simulink library "vil"  (Simulink 8.1)
settings: Solver=ode1  StartTime=0.0  StopTime=Inf  FixedStep=0.001  RelTol=1e-3
PostLoadFcn:
  | , if any(exist('dsrtsu_mdlpostloadfcn', 'file') == [2, 3, 6]), try dsrtsu_mdlpostloadfcn('Execute', bdroot); catch fprintf('Error in PostLoadFcn (dsrtsu_mdlpostloadfcn) for model "%s":\n %s\n', bdroot, lasterr); end, end,
undefined symbols (not defined in the file or in its folder): KIFO_VILOffsetToBumper_m
libraries: hcu_lib x1
settings Model: DSRTSU_INTERNAL_RTI_VER=450  DSRTSU_INTERNAL_RTI_TYPE=rti1401  RTICANMMDATA=struct('GeneralSetupData',struct('modelroot','D:\ELN150201_TAIWAN\trunk\AdasDragon\software\sw_development\arch\app\ifo','generalsettings',struct('filesettings',struct('destfolder',struct('Name','RTICANMM_FILES','Check',1),'buildfolder',struct('Name','.','Check',1),'AbsDestfolder',struct('Name','D:\ELN150201_TAIWAN\trunk\AdasDragon\software\sw_development\arch\app\ifo\RTICANMM_FILES'),'AbsBuildfolder',struct('Name','D:\ELN150201_TAIWAN\trunk\AdasDragon\software\sw_development\arch\app\ifo'))),'options',struct('addpaths',1,'rmpaths',1,'addtrcexclusion',logical(1),'cannavigator',struct('checkmonitoring',0),'show_usrtrc',0,'use_usrtrc',0),'advanced',struct('options',[1 1 1 1 1 1 1 1 1 1 1 1 1 1 1 1 1 1 1 1 1 1 1 1 1 1 1 1 1 1 1 1 1 1 1 1 1 1 1 1 1 1 1 1 1 1 1 1 1 1 1 1 1 1 1 1 1 1 1 1 1 1 1 1 1 1 1 1 1 1 1 1 1 1 1 1 1 1 1 1 1 1 1 1 1 1 1 1 1 1 1 1 1 1 1 1 1 1 1 1]),'MPSetup',{{}},'modelname','vil','block','vil'))  DSRTSU_INTERNAL_RTIFPGA=40  Creator=tescamilla  LastModifiedBy=AT015555

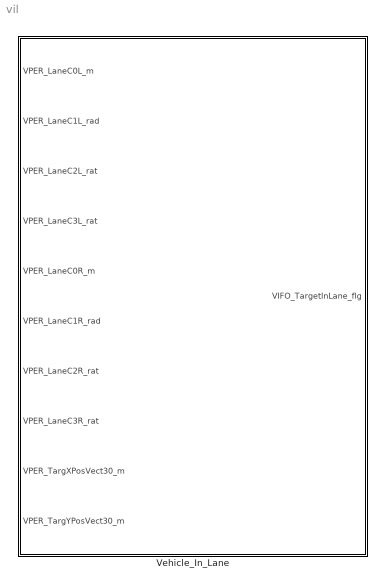
== system vil ==
  Vehicle_In_Lane : Subsystem

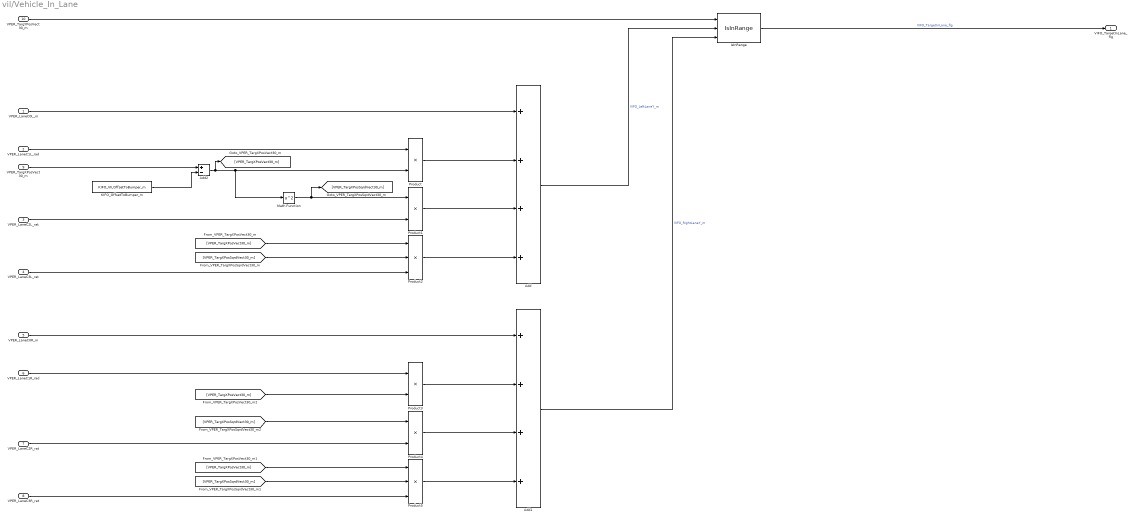
== system vil/Vehicle_In_Lane ==
  VPER_LaneC0L_m : Inport
  VPER_LaneC1L_rad : Inport  Port=2
  VPER_LaneC2L_rat : Inport  Port=3
  VPER_LaneC3L_rat : Inport  Port=4
  VPER_LaneC0R_m : Inport  Port=5
  VPER_LaneC1R_rad : Inport  Port=6
  VPER_LaneC2R_rat : Inport  Port=7
  VPER_LaneC3R_rat : Inport  Port=8
  VPER_TargXPosVect30_m : Inport  Port=9
  VPER_TargYPosVect30_m : Inport  Port=10
  Add : Sum  Inputs=++++
  Add1 : Sum  Inputs=++++
  Add2 : Sum  Inputs=+-
  IsInRange : hcu_lib/IsInRange  SystemSampleTime=-1
  KIFO_OffsetToBumper_m : Constant  Value=KIFO_VILOffsetToBumper_m
  Math Function : Math  Operator=square  SaturateOnIntegerOverflow=on
  Product{,1,3..4} (4 alike) : Product
  Product2 : Product  Inputs=3
  Product5 : Product  Inputs=3
  VIFO_TargetInLane_flg : Outport
  wires:
  VPER_LaneC1L_rad/1 -> Product/1
  Add2/1 -> [VPER_TargXPosVect30_m], Math Function/1, Product/2
  VPER_LaneC0L_m/1 -> Add/1
  Product/1 -> Add/2
  [VPER_TargXPosSqrdVect30_m] -> Product2/2
  VPER_LaneC2L_rat/1 -> Product1/2
  Product1/1 -> Add/3
  Math Function/1 -> [VPER_TargXPosSqrdVect30_m], Product1/1
  [VPER_TargXPosVect30_m] -> Product2/1
  VPER_LaneC3L_rat/1 -> Product2/3
  Product2/1 -> Add/4
  Add/1 -> IsInRange/2  "VIFO_LeftLaneY_m"
  VPER_LaneC0R_m/1 -> Add1/1
  VPER_LaneC1R_rad/1 -> Product3/1
  Product3/1 -> Add1/2
  [VPER_TargXPosVect30_m] -> Product3/2
  VPER_LaneC2R_rat/1 -> Product4/2
  Product4/1 -> Add1/3
  [VPER_TargXPosSqrdVect30_m] -> Product5/2
  [VPER_TargXPosVect30_m] -> Product5/1
  VPER_LaneC3R_rat/1 -> Product5/3
  Product5/1 -> Add1/4
  Add1/1 -> IsInRange/3  "VIFO_RightLaneY_m"
  [VPER_TargXPosSqrdVect30_m] -> Product4/1
  VPER_TargYPosVect30_m/1 -> IsInRange/1
  IsInRange/1 -> VIFO_TargetInLane_flg/1  "VIFO_TargetInLane_flg"
  VPER_TargXPosVect30_m/1 -> Add2/1
  KIFO_OffsetToBumper_m/1 -> Add2/2
